simulink library "Power_Calc_Lib"  (R2024a)
settings: Solver=VariableStepAuto  StartTime=0.0  StopTime=10.0  RelTol=1e-3
undefined symbols (not defined in the file): Newton, Raphson
libraries: spsRMSLib x10, spsFourierLib x2, spsMeanLib x2
Description:
  | Copyright 2019-2024 The MathWorks, Inc.
settings Model: Creator=smiller  LastModifiedBy=smiller
settings SolverCC: AlgebraicLoopSolver=TrustRegion
settings OptimizationCC: ReuseModelBlockBuffer=off
settings DebuggingCC: UnconnectedInputMsg=warning  UnconnectedOutputMsg=warning  UnconnectedLineMsg=warning
settings ModelReferenceCC: EnableRefExpFcnMdlSchedulingChecks=on
settings SFSimCC: CustomCodeUndefinedFunction=UseInterfaceOnly
settings RTWCC: GPUComputeCapability=3.5  DLArmComputeVersion=19.05

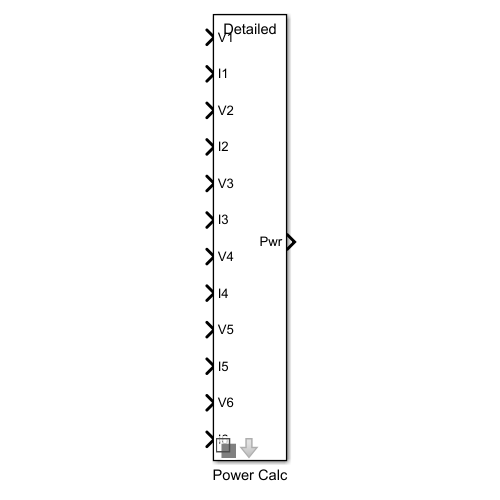
[thumbnail: Simulink's stored preview of the top-level diagram]
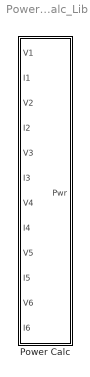
== system Power_Calc_Lib ==
  Power Calc : Subsystem  Variant=on  VariantControlMode=label  LabelModeActiveChoice=Detailed  mask{ModelType=Detailed}
      mask prompts: ModelType "Model Type"
      mask init:
      | set_param(gcb,'LabelModeActiveChoice',get_param(gcb,'ModelType'));
      settings: AttributesFormatString=%<BlockChoice>
      mask TypeOptions ModelType: Detailed | Phasor

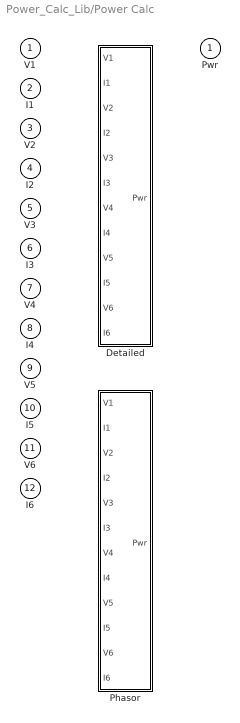
== system Power_Calc_Lib/Power Calc ==
  V1 : Inport
  I1 : Inport  Port=2
  V2 : Inport  Port=3
  I2 : Inport  Port=4
  V3 : Inport  Port=5
  I3 : Inport  Port=6
  V4 : Inport  Port=7
  I4 : Inport  Port=8
  V5 : Inport  Port=9
  I5 : Inport  Port=10
  V6 : Inport  Port=11
  I6 : Inport  Port=12
  Detailed : Subsystem  VariantControl=Detailed
  Phasor : Subsystem  VariantControl=Phasor
  Pwr : Outport  VectorParamsAs1DForOutWhenUnconnected=off

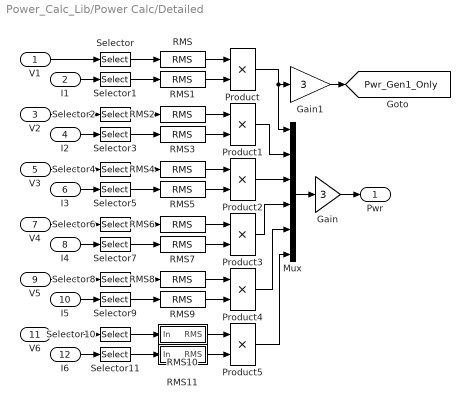
== system Power_Calc_Lib/Power Calc/Detailed ==
  V1 : Inport
  I1 : Inport  Port=2
  V2 : Inport  Port=3
  I2 : Inport  Port=4
  V3 : Inport  Port=5
  I3 : Inport  Port=6
  V4 : Inport  Port=7
  I4 : Inport  Port=8
  V5 : Inport  Port=9
  I5 : Inport  Port=10
  V6 : Inport  Port=11
  I6 : Inport  Port=12
  Gain : Gain  Gain=3
  Gain1 : Gain  Gain=3
  Mux : Mux  Inputs=6
  Product{,1..5} (6 alike) : Product
  RMS{,1..9} (10 alike) : spsRMSLib/RMS  TrueRMS=on  Freq=400  RMSInit=0  Ts=0
  RMS10 : Subsystem  DialogController=POWERSYS.PowerSysDialog  mask(RMS){TrueRMS=on, Freq=400, RMSInit=0, Ts=0}
      mask prompts: TrueRMS "True RMS value"; Freq "Fundamental frequency (Hz):"; RMSInit "Initial RMS value:"; Ts "Sample time:"
      mask help:
      | Measure the true root mean square (RMS) value of the input signal at the specified fundamental frequency.
      |
      | When True RMS value parameter is unchecked, the block outputs the RMS value of the fundamental component of the input signal.
      mask init:
      | [sps] = powericon('RMSInit',gcb,Freq,RMSInit,TrueRMS,Ts);
      mask Help: helpview(psbhelp);
      mask Display: color('blue');disp('RMS')
  RMS11 : Subsystem  DialogController=POWERSYS.PowerSysDialog  mask(RMS){TrueRMS=on, Freq=400, RMSInit=0, Ts=0}
      mask prompts: TrueRMS "True RMS value"; Freq "Fundamental frequency (Hz):"; RMSInit "Initial RMS value:"; Ts "Sample time:"
      mask help:
      | Measure the true root mean square (RMS) value of the input signal at the specified fundamental frequency.
      |
      | When True RMS value parameter is unchecked, the block outputs the RMS value of the fundamental component of the input signal.
      mask init:
      | [sps] = powericon('RMSInit',gcb,Freq,RMSInit,TrueRMS,Ts);
      mask Help: helpview(psbhelp);
      mask Display: color('blue');disp('RMS')
  Selector{,1..11} (12 alike) : Selector  InputPortWidth=3  IndexOptions=Index vector (dialog)  Indices=[1]  OutputSizes=1
  Pwr : Outport  VectorParamsAs1DForOutWhenUnconnected=off
  tag scope: Pwr_Gen1_Only=global
  wires:
  RMS8/1 -> Product4/1
  RMS9/1 -> Product4/2
  V5/1 -> Selector8/1
  I5/1 -> Selector9/1
  V4/1 -> Selector6/1
  RMS6/1 -> Product3/1
  I4/1 -> Selector7/1
  RMS7/1 -> Product3/2
  RMS4/1 -> Product2/1
  I3/1 -> Selector5/1
  V3/1 -> Selector4/1
  RMS5/1 -> Product2/2
  RMS2/1 -> Product1/1
  I2/1 -> Selector3/1
  RMS3/1 -> Product1/2
  V2/1 -> Selector2/1
  RMS/1 -> Product/1
  RMS1/1 -> Product/2
  Product/1 -> Gain1/1, Mux/1
  Product3/1 -> Mux/4
  Product2/1 -> Mux/3
  Product1/1 -> Mux/2
  Product4/1 -> Mux/5
  Mux/1 -> Gain/1
  V1/1 -> Selector/1
  I1/1 -> Selector1/1
  Selector/1 -> RMS/1
  Selector1/1 -> RMS1/1
  Selector2/1 -> RMS2/1
  Selector3/1 -> RMS3/1
  Selector4/1 -> RMS4/1
  Selector5/1 -> RMS5/1
  Selector6/1 -> RMS6/1
  Selector7/1 -> RMS7/1
  Selector8/1 -> RMS8/1
  Selector9/1 -> RMS9/1
  Gain/1 -> Pwr/1
  RMS10/1(RMS) -> Product5/1
  RMS11/1(RMS) -> Product5/2
  V6/1 -> Selector10/1
  I6/1 -> Selector11/1
  Selector10/1 -> RMS10/1(In)
  Selector11/1 -> RMS11/1(In)
  Product5/1 -> Mux/6
  Gain1/1 -> [Pwr_Gen1_Only]

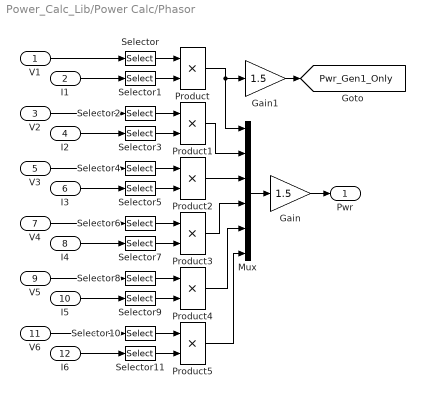
== system Power_Calc_Lib/Power Calc/Phasor ==
  V1 : Inport
  I1 : Inport  Port=2
  V2 : Inport  Port=3
  I2 : Inport  Port=4
  V3 : Inport  Port=5
  I3 : Inport  Port=6
  V4 : Inport  Port=7
  I4 : Inport  Port=8
  V5 : Inport  Port=9
  I5 : Inport  Port=10
  V6 : Inport  Port=11
  I6 : Inport  Port=12
  Gain : Gain  Gain=1.5
  Gain1 : Gain  Gain=1.5
  Mux : Mux  Inputs=6
  Product{,1..5} (6 alike) : Product
  Selector{,1..11} (12 alike) : Selector  InputPortWidth=3  IndexOptions=Index vector (dialog)  Indices=[1]  OutputSizes=1
  Pwr : Outport  VectorParamsAs1DForOutWhenUnconnected=off
  tag scope: Pwr_Gen1_Only=global
  wires:
  Mux/1 -> Gain/1
  Product4/1 -> Mux/5
  Product1/1 -> Mux/2
  Product2/1 -> Mux/3
  Product3/1 -> Mux/4
  Product/1 -> Gain1/1, Mux/1
  I1/1 -> Selector1/1
  V1/1 -> Selector/1
  I2/1 -> Selector3/1
  V2/1 -> Selector2/1
  I3/1 -> Selector5/1
  V3/1 -> Selector4/1
  I4/1 -> Selector7/1
  V4/1 -> Selector6/1
  I5/1 -> Selector9/1
  V5/1 -> Selector8/1
  Gain/1 -> Pwr/1
  Selector/1 -> Product/1
  Selector1/1 -> Product/2
  Selector2/1 -> Product1/1
  Selector3/1 -> Product1/2
  Selector4/1 -> Product2/1
  Selector5/1 -> Product2/2
  Selector6/1 -> Product3/1
  Selector7/1 -> Product3/2
  Selector8/1 -> Product4/1
  Selector9/1 -> Product4/2
  I6/1 -> Selector11/1
  V6/1 -> Selector10/1
  Selector10/1 -> Product5/1
  Selector11/1 -> Product5/2
  Product5/1 -> Mux/6
  Gain1/1 -> [Pwr_Gen1_Only]

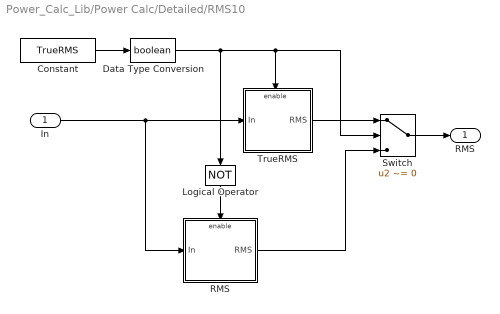
== system Power_Calc_Lib/Power Calc/Detailed/RMS10 ==
  In : Inport  SampleTime=Ts
  Constant : Constant  Value=TrueRMS
  Data Type Conversion : DataTypeConversion  OutDataTypeStr=boolean  SaturateOnIntegerOverflow=off  RndMeth=Floor
  Logical Operator : Logic  Operator=NOT  AllPortsSameDT=off  OutDataTypeStr=boolean
  "RMS " : Subsystem
  Switch : Switch  Criteria=u2 ~= 0  Threshold=0.5  SaturateOnIntegerOverflow=off  InputSameDT=off
  "TrueRMS " : Subsystem
  RMS : Outport  SampleTime=Ts  VectorParamsAs1DForOutWhenUnconnected=off
  wires:
  Logical Operator/1 -> "RMS "/Enable
  Data Type Conversion/1 -> Switch/2, "TrueRMS "/Enable, Logical Operator/1
  Constant/1 -> Data Type Conversion/1
  "RMS "/1(RMS) -> Switch/3
  "TrueRMS "/1(RMS) -> Switch/1
  Switch/1 -> RMS/1
  In/1 -> "RMS "/1(In), "TrueRMS "/1(In)

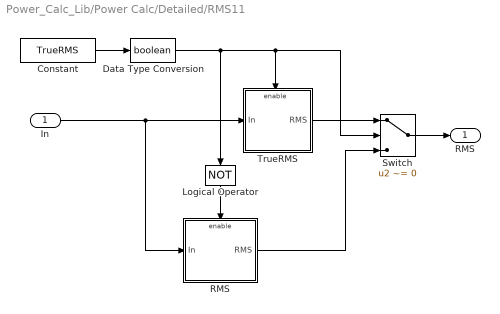
== system Power_Calc_Lib/Power Calc/Detailed/RMS11 ==
  In : Inport  SampleTime=Ts
  Constant : Constant  Value=TrueRMS
  Data Type Conversion : DataTypeConversion  OutDataTypeStr=boolean  SaturateOnIntegerOverflow=off  RndMeth=Floor
  Logical Operator : Logic  Operator=NOT  AllPortsSameDT=off  OutDataTypeStr=boolean
  "RMS " : Subsystem
  Switch : Switch  Criteria=u2 ~= 0  Threshold=0.5  SaturateOnIntegerOverflow=off  InputSameDT=off
  "TrueRMS " : Subsystem
  RMS : Outport  SampleTime=Ts  VectorParamsAs1DForOutWhenUnconnected=off
  wires:
  Logical Operator/1 -> "RMS "/Enable
  Data Type Conversion/1 -> Switch/2, "TrueRMS "/Enable, Logical Operator/1
  Constant/1 -> Data Type Conversion/1
  "RMS "/1(RMS) -> Switch/3
  "TrueRMS "/1(RMS) -> Switch/1
  Switch/1 -> RMS/1
  In/1 -> "RMS "/1(In), "TrueRMS "/1(In)

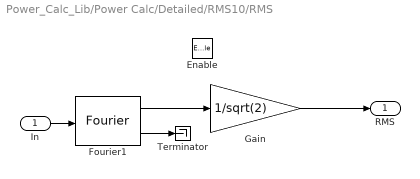
== system Power_Calc_Lib/Power Calc/Detailed/RMS10/RMS  ==
  In : Inport
  Enable : EnablePort
  Fourier1 : spsFourierLib/Fourier  Freq=sps.Freq  n=1  InInit=[0 0]  Ts=Ts
  Gain : Gain  Gain=1/sqrt(2)
  Terminator : Terminator
  RMS : Outport  VectorParamsAs1DForOutWhenUnconnected=off
  wires:
  Gain/1 -> RMS/1
  In/1 -> Fourier1/1
  Fourier1/2 -> Terminator/1
  Fourier1/1 -> Gain/1

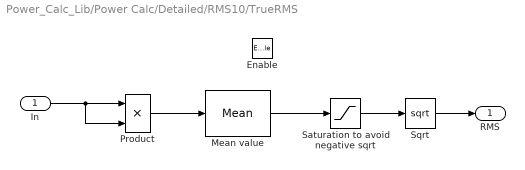
== system Power_Calc_Lib/Power Calc/Detailed/RMS10/TrueRMS  ==
  In : Inport
  Enable : EnablePort
  Mean value : spsMeanLib/Mean  Freq=sps.Freq  Vinit=sps.Par_Init_TrueRMS  Ts=Ts
  Product : Product  InputSameDT=on  SaturateOnIntegerOverflow=on  OutDataTypeStr=Inherit: Same as first input
  Saturation to avoid negative sqrt : Saturate  UpperLimit=Inf  LowerLimit=0
  Sqrt : Sqrt  AlgorithmType=Newton-Raphson
  RMS : Outport  VectorParamsAs1DForOutWhenUnconnected=off
  wires:
  Sqrt/1 -> RMS/1
  In/1 -> Product/1, Product/2
  Product/1 -> Mean value/1
  Mean value/1 -> Saturation to avoid negative sqrt/1
  Saturation to avoid negative sqrt/1 -> Sqrt/1

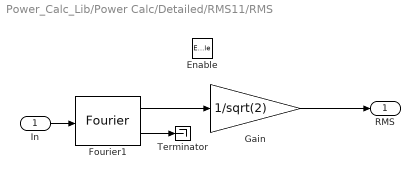
== system Power_Calc_Lib/Power Calc/Detailed/RMS11/RMS  ==
  In : Inport
  Enable : EnablePort
  Fourier1 : spsFourierLib/Fourier  Freq=sps.Freq  n=1  InInit=[0 0]  Ts=Ts
  Gain : Gain  Gain=1/sqrt(2)
  Terminator : Terminator
  RMS : Outport  VectorParamsAs1DForOutWhenUnconnected=off
  wires:
  Gain/1 -> RMS/1
  In/1 -> Fourier1/1
  Fourier1/2 -> Terminator/1
  Fourier1/1 -> Gain/1

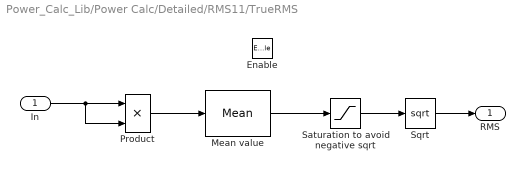
== system Power_Calc_Lib/Power Calc/Detailed/RMS11/TrueRMS  ==
  In : Inport
  Enable : EnablePort
  Mean value : spsMeanLib/Mean  Freq=sps.Freq  Vinit=sps.Par_Init_TrueRMS  Ts=Ts
  Product : Product  InputSameDT=on  SaturateOnIntegerOverflow=on  OutDataTypeStr=Inherit: Same as first input
  Saturation to avoid negative sqrt : Saturate  UpperLimit=Inf  LowerLimit=0
  Sqrt : Sqrt  AlgorithmType=Newton-Raphson
  RMS : Outport  VectorParamsAs1DForOutWhenUnconnected=off
  wires:
  Sqrt/1 -> RMS/1
  In/1 -> Product/1, Product/2
  Product/1 -> Mean value/1
  Mean value/1 -> Saturation to avoid negative sqrt/1
  Saturation to avoid negative sqrt/1 -> Sqrt/1
